simulink model "testmodel"  (R2025b)
settings: Solver=VariableStepAuto  StartTime=0.0  StopTime=2  RelTol=1e-3
libraries: audiofeatures x2, audiosources x1, statsLibrary x1, deeplib x1
settings Model: Creator=prashanth  LastModifiedBy=prashanth

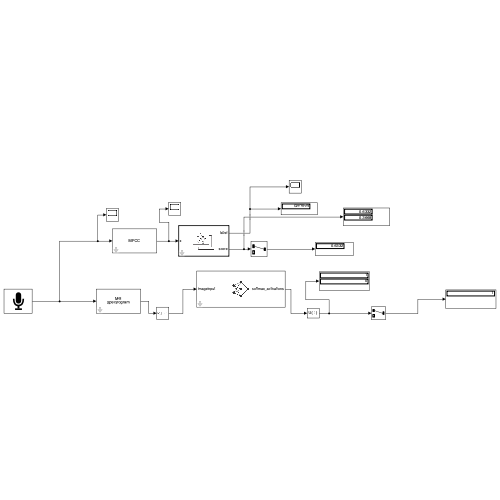
[thumbnail: Simulink's stored preview of the top-level diagram]
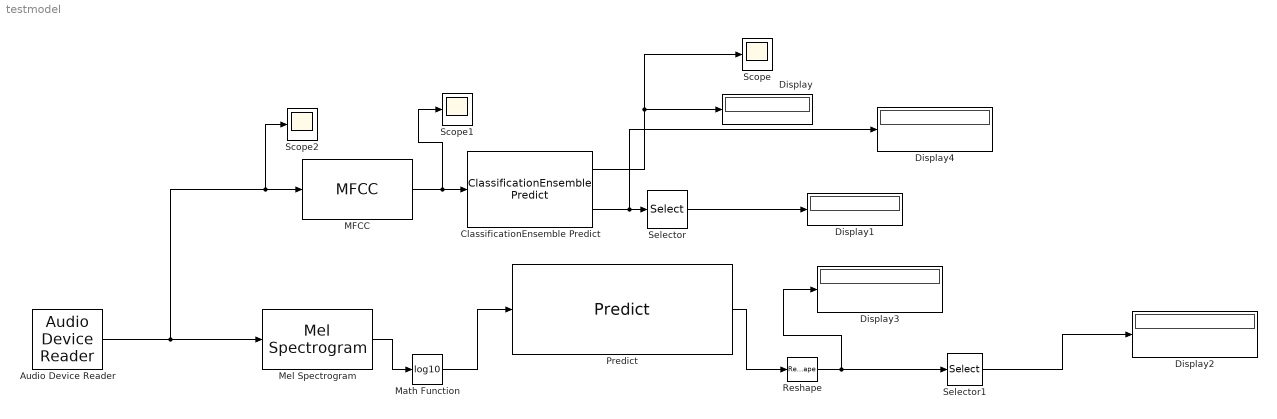
== system testmodel ==
  Audio Device Reader : audiosources/Audio Device Reader  Driver=CoreAudio  Device=Default  SampleRate=44100  NumChannels=1  SamplesPerFrame=44100  BitDepth=16-bit integer  NumBuffers=10  DefaultInputChannelMapping=on  InputChannelMapping=1:2  OutputNumOverrunSamples=off  OutputDataType=double  DriverIdx=5  DeviceWarnFlag=''
  ClassificationEnsemble Predict : statsLibrary/Classification/ClassificationEnsemble Predict  TrainedLearner=trainedModel  ShowOutputScore=on  LabelOutMin=[]  LabelOutMax=[]  ScoreOutMin=[]  ScoreOutMax=[]  RawScoreOutMin=[]  RawScoreOutMax=[]  WeakLearnerOutMin=[]  WeakLearnerOutMax=[]  StoredEnumName=trainedModel_enumLabels
  Display{,1..4} (5 alike) : Display
  MFCC : audiofeatures/MFCC  WindowParameter=hamming(1024,'periodic')  OverlapLength=512  NumCoeffs=13  Rectification=Logarithm  AppendDelta=on  AppendDeltaDelta=off  DeltaWindowLength=9  NumFeatureVectors=1  NumFeatureVectorOverlap=0  InheritSampleRate=on  SampleRate=44.1e3  NumBands=32  AutoFrequencyRange=on  FrequencyRange=[0, 22050]  FilterBankDesignDomain=linear  FilterBankNormalization=bandwidth  MelStyle=oshaughnessy  WindowNormalization=on  SpectrumType=power  AutoFFTLength=on  FFTLength=1024
  Math Function : Math  Operator=log10
  Mel Spectrogram : audiofeatures/Mel Spectrogram  FrequencyScale=mel  AutoNumBands=off  NumBands=32  AutoFrequencyRange=on  FrequencyRange=[0, 22050]  FilterBankDesignDomain=linear  FilterBankNormalization=bandwidth  MelStyle=oshaughnessy  OutputFrequencyVector=off  WindowParameter=hamming(1024,'periodic')  WindowNormalization=on  OverlapLength=512  AutoFFTLength=on  FFTLength=1024  SpectrumType=magnitude  ApplyLog=off  NumHops=85  NumHopsOverlap=0  InheritSampleRate=on  SampleRate=44.1e3
  Predict : deeplib/Predict  Network=Network from MAT-file  NetworkFunction=squeezenet  NetworkFilePath=/Users/prashanth/Desktop/karthik/gunshotCNN.mat  MiniBatchSize=128  InputDataFormats={'',''}  Predictions=off  Activations={'softmax'}  ForceInterpretedSim=off  EnableDLNetwork=on  LastKnownNetworkFilePath=''  LastKnownNetworkTimeStamp=''
  Reshape : Reshape
  Scope : Scope
      settings: ActiveDisplayYMinimum=-1  ActiveDisplayYMaximum=1
  Scope1 : Scope
      settings: ActiveDisplayYMinimum=-1  ActiveDisplayYMaximum=1
  Scope2 : Scope
      settings: ActiveDisplayYMinimum=-0.023110870089254609  ActiveDisplayYMaximum=0.0453552937613908  DataLoggingVariableName=ScopeData2
  Selector : Selector  InputPortWidth=2  IndexOptions=Index vector (dialog)  Indices=1  OutputSizes=1
  Selector1 : Selector  InputPortWidth=2  IndexOptions=Index vector (dialog)  Indices=1  OutputSizes=1
  wires:
  MFCC/1 -> Scope1/1, ClassificationEnsemble Predict/1
  ClassificationEnsemble Predict/1 -> Scope/1, Display/1
  ClassificationEnsemble Predict/2 -> Display4/1, Selector/1
  Selector/1 -> Display1/1
  Audio Device Reader/1 -> Scope2/1, MFCC/1, Mel Spectrogram/1
  Mel Spectrogram/1 -> Math Function/1
  Math Function/1 -> Predict/1
  Predict/1 -> Reshape/1
  Reshape/1 -> Selector1/1, Display3/1
  Selector1/1 -> Display2/1
